simulink model "filterbankFIRFINALNOCOMP"  (R2018a)
settings: Solver=FixedStepDiscrete  StartTime=0.0  StopTime=0.001  RelTol=1e-3
values from neighbouring files (symbols this model uses):
  fs = 20000    [filterbankProto.m]    (also in main.m = 44100)
  gainConsts = 10.^(requiredGainDB/10)    [main.m]
undefined symbols (not defined in the file or in its folder): fdesignblkfcn, gcbh
libraries: dspsrcs4 x1, dspxfrm3 x1, dspobslib x1
(part 1 of 3)
settings Model: SimulationMode=accelerator  Creator=Kavi  LastModifiedBy=Kavi
settings SolverCC: AutoInsertRateTranBlk=on
settings DataIOCC: LimitDataPoints=on  SaveOutput=off  SignalLogging=off  SaveTime=off
settings OptimizationCC: LifeSpan=inf  SimCompilerOptimization=on
settings DebuggingCC: AlgebraicLoopMsg=error  SingleTaskRateTransMsg=error  AllowSymbolicDim=off  SFUnexpectedBacktrackingDiag=warning  SFNoUnconditionalDefaultTransitionDiag=warning  SFExecutionAtInitializationDiag=none
settings CodeAppCC: StateflowObjectComments=on
settings GRTTargetCC: TargetLangStandard=C89/C90 (ANSI)  GeneratePreprocessorConditionals=Disable all
settings ConfigComp: CovMetricSettings=dw  CovHtmlReporting=on  CovSaveCumulativeToWorkspaceVar=on  CovSaveSingleToWorkspaceVar=on  CovExternalEMLEnable=off  CovSFcnEnable=off

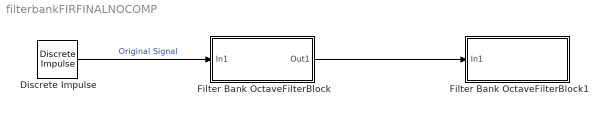
== system filterbankFIRFINALNOCOMP ==
  Discrete Impulse : dspsrcs4/Discrete  Impulse  Delay=0  SampleTime=1/fs  FrameSample=512  OutputFrames=off  dataType=double  isSigned=on  wordLen=16  udDataType=sfix(16)  fracBitsMode=Best precision  numFracBits=15  OutDataTypeStr=double  LastOutDataTypeStr=double
  Filter Bank OctaveFilterBlock : Subsystem
  Filter Bank OctaveFilterBlock1 : Subsystem
  wires:
  Discrete Impulse/1 -> Filter Bank OctaveFilterBlock/1(In1)  "Original Signal"
  Filter Bank OctaveFilterBlock/1(Out1) -> Filter Bank OctaveFilterBlock1/1(In1)

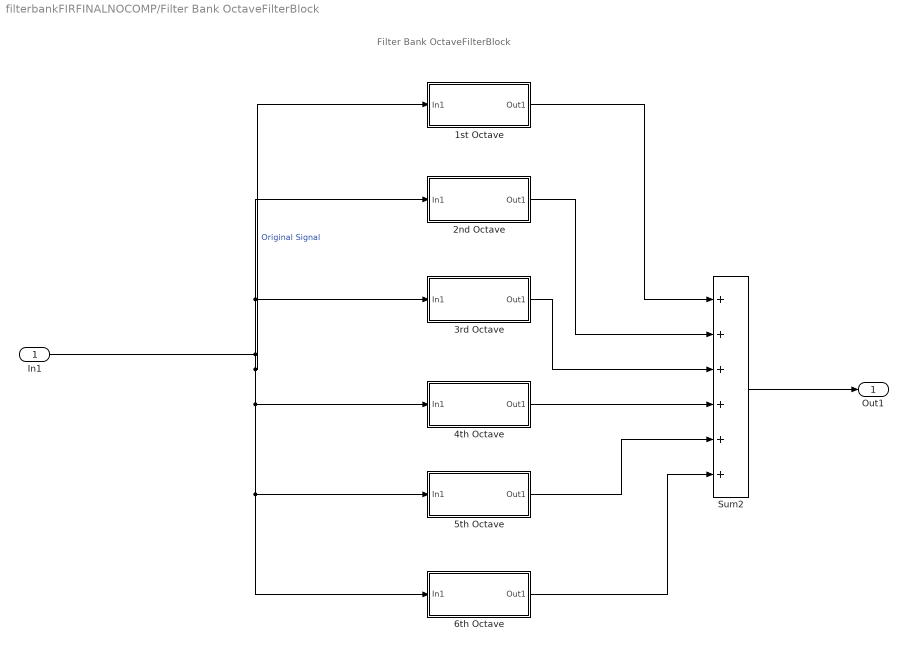
== system filterbankFIRFINALNOCOMP/Filter Bank OctaveFilterBlock ==
  note: Filter Bank OctaveFilterBlock
  In1 : Inport
  "1st Octave " : Subsystem
  2nd Octave : Subsystem
  "3rd Octave " : Subsystem
  4th Octave : Subsystem
  5th Octave : Subsystem
  6th Octave : Subsystem
  Sum2 : Sum  Inputs=++++++
  Out1 : Outport
  wires:
  Sum2/1 -> Out1/1
  2nd Octave/1(Out1) -> Sum2/2
  "3rd Octave "/1(Out1) -> Sum2/3
  4th Octave/1(Out1) -> Sum2/4
  5th Octave/1(Out1) -> Sum2/5
  6th Octave/1(Out1) -> Sum2/6
  In1/1 -> 4th Octave/1(In1), 5th Octave/1(In1), 6th Octave/1(In1), "1st Octave "/1(In1), "3rd Octave "/1(In1), 2nd Octave/1(In1)  "Original Signal"
  "1st Octave "/1(Out1) -> Sum2/1

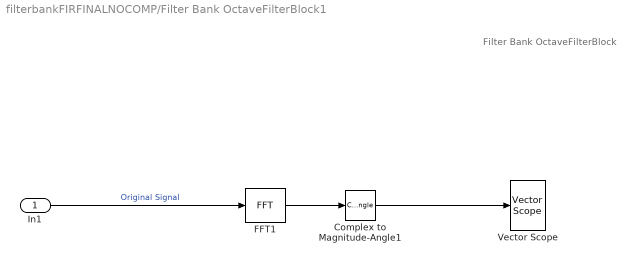
== system filterbankFIRFINALNOCOMP/Filter Bank OctaveFilterBlock1 ==
  note: Filter Bank OctaveFilterBlock
  In1 : Inport
  Complex to Magnitude-Angle1 : ComplexToMagnitudeAngle  Output=Magnitude
  FFT1 : dspxfrm3/FFT  FFTImplementation=Auto  CompMethod=Table lookup  TableOpt=NEW  TableOptActive=Speed  BitRevOrder=off  Normalize=off  InheritFFTLength=on  FFTLength=64  WrapInput=on  roundingMode=Floor  overflowMode=off  firstCoeffDataTypeStr=Inherit: Same word length as input  firstCoeffLastDataTypeStr=Inherit: Same word length as input  outputMin=[]  outputMax=[]
  Vector Scope : dspobslib/Vector Scope  ScopeProperties=off  Domain=Frequency  HorizSpan=1  DisplayProperties=off  AxisGrid=on  Memory=off  FrameNumber=on  AxisLegend=off  AxisZoom=off  OpenScopeAtSimStart=on  OpenScopeImmediately=off  FigPos=[86 244 1118 420]  AxisProperties=on  XUnits=Hertz  XRange=[0...Fs/2]  InheritXIncr=on  XIncr=1  XLabel=Samples  XLimit=Auto  XMin=0  XMax=1  XStart=0  YUnits=dB  YLabel=|Magnitude (dB)|  LineProperties=off  LineStyles=-  LineMarkers=None  LineColors=[0 0 0]  XAxisParamsVer=6.9
      settings: SourceProductName=DSP System Toolbox  SourceProductBaseCode=DS  YMin=0.0723692553519949  YMax=69.3188381671759
  wires:
  Complex to Magnitude-Angle1/1 -> Vector Scope/1
  FFT1/1 -> Complex to Magnitude-Angle1/1
  In1/1 -> FFT1/1  "Original Signal"

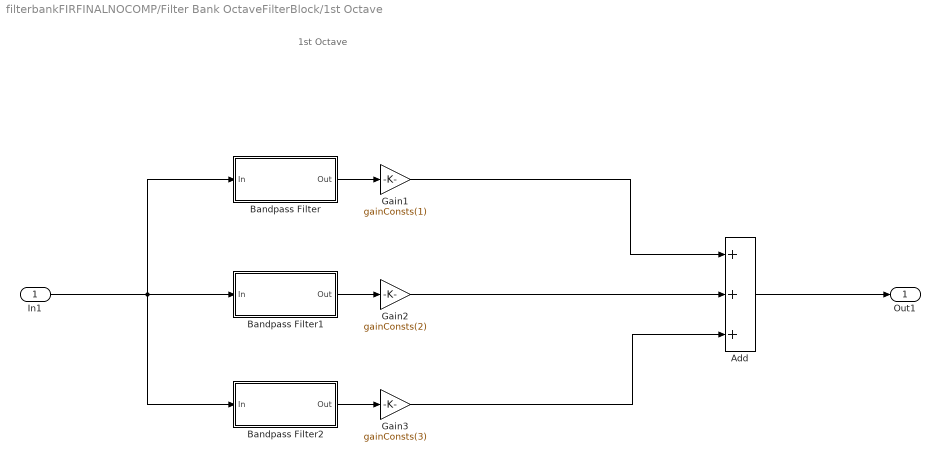
== system filterbankFIRFINALNOCOMP/Filter Bank OctaveFilterBlock/1st Octave  ==
  note: 1st Octave
  In1 : Inport
  Add : Sum  Inputs=+++
  Bandpass Filter : Subsystem  DialogController=fdesignblkfcn  InitFcn=fdesignblkfcn(gcbh, {'InitFcn'});  mask(Bandpass Filter){}
      mask help: Design a bandpass filter
      settings: CopyFcn=fdesignblkfcn(gcbh, {'CopyFcn'});
      mask Help: helpview(mapfilelocation('dsp'), 'dspbandpassfilter');
      mask Display: disp('Bandpass');
  Bandpass Filter1 : Subsystem  DialogController=fdesignblkfcn  InitFcn=fdesignblkfcn(gcbh, {'InitFcn'});  mask(Bandpass Filter){}
      mask help: Design a bandpass filter
      settings: CopyFcn=fdesignblkfcn(gcbh, {'CopyFcn'});
      mask Help: helpview(mapfilelocation('dsp'), 'dspbandpassfilter');
      mask Display: disp('Bandpass');
  Bandpass Filter2 : Subsystem  DialogController=fdesignblkfcn  InitFcn=fdesignblkfcn(gcbh, {'InitFcn'});  mask(Bandpass Filter){}
      mask help: Design a bandpass filter
      settings: CopyFcn=fdesignblkfcn(gcbh, {'CopyFcn'});
      mask Help: helpview(mapfilelocation('dsp'), 'dspbandpassfilter');
      mask Display: disp('Bandpass');
  Gain1 : Gain  Gain=gainConsts(1)
  Gain2 : Gain  Gain=gainConsts(2)
  Gain3 : Gain  Gain=gainConsts(3)
  Out1 : Outport
  wires:
  Bandpass Filter1/1(Out) -> Gain2/1
  Bandpass Filter2/1(Out) -> Gain3/1
  Add/1 -> Out1/1
  In1/1 -> Bandpass Filter/1(In), Bandpass Filter2/1(In), Bandpass Filter1/1(In)
  Bandpass Filter/1(Out) -> Gain1/1
  Gain1/1 -> Add/1
  Gain2/1 -> Add/2
  Gain3/1 -> Add/3

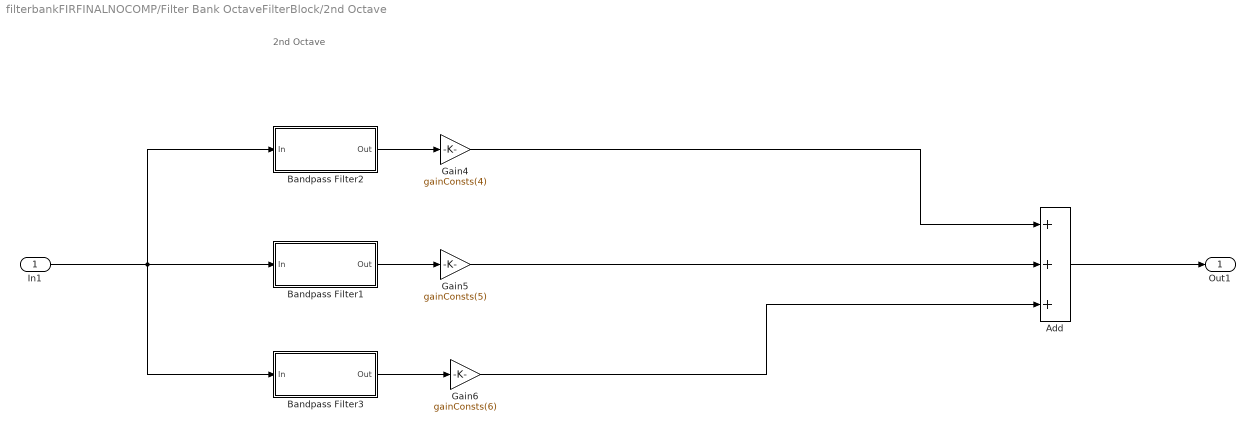
== system filterbankFIRFINALNOCOMP/Filter Bank OctaveFilterBlock/2nd Octave ==
  note: 2nd Octave
  In1 : Inport
  Add : Sum  Inputs=+++
  Bandpass Filter1 : Subsystem  DialogController=fdesignblkfcn  InitFcn=fdesignblkfcn(gcbh, {'InitFcn'});  mask(Bandpass Filter){}
      mask help: Design a bandpass filter
      settings: CopyFcn=fdesignblkfcn(gcbh, {'CopyFcn'});
      mask Help: helpview(mapfilelocation('dsp'), 'dspbandpassfilter');
      mask Display: disp('Bandpass');
  Bandpass Filter2 : Subsystem  DialogController=fdesignblkfcn  InitFcn=fdesignblkfcn(gcbh, {'InitFcn'});  mask(Bandpass Filter){}
      mask help: Design a bandpass filter
      settings: CopyFcn=fdesignblkfcn(gcbh, {'CopyFcn'});
      mask Help: helpview(mapfilelocation('dsp'), 'dspbandpassfilter');
      mask Display: disp('Bandpass');
  Bandpass Filter3 : Subsystem  DialogController=fdesignblkfcn  InitFcn=fdesignblkfcn(gcbh, {'InitFcn'});  mask(Bandpass Filter){}
      mask help: Design a bandpass filter
      settings: CopyFcn=fdesignblkfcn(gcbh, {'CopyFcn'});
      mask Help: helpview(mapfilelocation('dsp'), 'dspbandpassfilter');
      mask Display: disp('Bandpass');
  Gain4 : Gain  Gain=gainConsts(4)
  Gain5 : Gain  Gain=gainConsts(5)
  Gain6 : Gain  Gain=gainConsts(6)
  Out1 : Outport
  wires:
  In1/1 -> Bandpass Filter3/1(In), Bandpass Filter1/1(In), Bandpass Filter2/1(In)
  Bandpass Filter1/1(Out) -> Gain5/1
  Bandpass Filter2/1(Out) -> Gain4/1
  Bandpass Filter3/1(Out) -> Gain6/1
  Add/1 -> Out1/1
  Gain4/1 -> Add/1
  Gain5/1 -> Add/2
  Gain6/1 -> Add/3

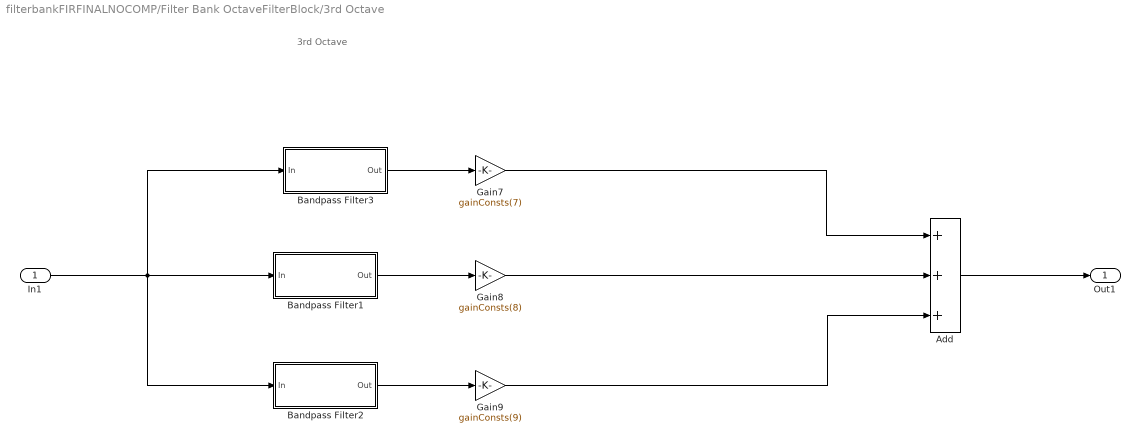
== system filterbankFIRFINALNOCOMP/Filter Bank OctaveFilterBlock/3rd Octave  ==
  note: 3rd Octave
  In1 : Inport
  Add : Sum  Inputs=+++
  Bandpass Filter1 : Subsystem  DialogController=fdesignblkfcn  InitFcn=fdesignblkfcn(gcbh, {'InitFcn'});  mask(Bandpass Filter){}
      mask help: Design a bandpass filter
      settings: CopyFcn=fdesignblkfcn(gcbh, {'CopyFcn'});
      mask Help: helpview(mapfilelocation('dsp'), 'dspbandpassfilter');
      mask Display: disp('Bandpass');
  Bandpass Filter2 : Subsystem  DialogController=fdesignblkfcn  InitFcn=fdesignblkfcn(gcbh, {'InitFcn'});  mask(Bandpass Filter){}
      mask help: Design a bandpass filter
      settings: CopyFcn=fdesignblkfcn(gcbh, {'CopyFcn'});
      mask Help: helpview(mapfilelocation('dsp'), 'dspbandpassfilter');
      mask Display: disp('Bandpass');
  Bandpass Filter3 : Subsystem  DialogController=fdesignblkfcn  InitFcn=fdesignblkfcn(gcbh, {'InitFcn'});  mask(Bandpass Filter){}
      mask help: Design a bandpass filter
      settings: CopyFcn=fdesignblkfcn(gcbh, {'CopyFcn'});
      mask Help: helpview(mapfilelocation('dsp'), 'dspbandpassfilter');
      mask Display: disp('Bandpass');
  Gain7 : Gain  Gain=gainConsts(7)
  Gain8 : Gain  Gain=gainConsts(8)
  Gain9 : Gain  Gain=gainConsts(9)
  Out1 : Outport
  wires:
  In1/1 -> Bandpass Filter2/1(In), Bandpass Filter1/1(In), Bandpass Filter3/1(In)
  Bandpass Filter1/1(Out) -> Gain8/1
  Bandpass Filter3/1(Out) -> Gain7/1
  Bandpass Filter2/1(Out) -> Gain9/1
  Add/1 -> Out1/1
  Gain7/1 -> Add/1
  Gain8/1 -> Add/2
  Gain9/1 -> Add/3

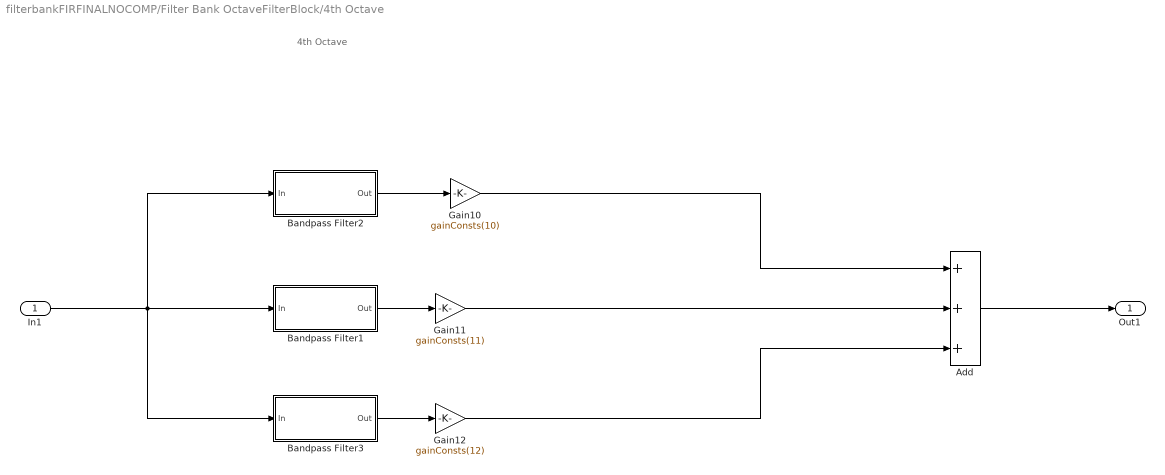
== system filterbankFIRFINALNOCOMP/Filter Bank OctaveFilterBlock/4th Octave ==
  note: 4th Octave
  In1 : Inport
  Add : Sum  Inputs=+++
  Bandpass Filter1 : Subsystem  DialogController=fdesignblkfcn  InitFcn=fdesignblkfcn(gcbh, {'InitFcn'});  mask(Bandpass Filter){}
      mask help: Design a bandpass filter
      settings: CopyFcn=fdesignblkfcn(gcbh, {'CopyFcn'});
      mask Help: helpview(mapfilelocation('dsp'), 'dspbandpassfilter');
      mask Display: disp('Bandpass');
  Bandpass Filter2 : Subsystem  DialogController=fdesignblkfcn  InitFcn=fdesignblkfcn(gcbh, {'InitFcn'});  mask(Bandpass Filter){}
      mask help: Design a bandpass filter
      settings: CopyFcn=fdesignblkfcn(gcbh, {'CopyFcn'});
      mask Help: helpview(mapfilelocation('dsp'), 'dspbandpassfilter');
      mask Display: disp('Bandpass');
  Bandpass Filter3 : Subsystem  DialogController=fdesignblkfcn  InitFcn=fdesignblkfcn(gcbh, {'InitFcn'});  mask(Bandpass Filter){}
      mask help: Design a bandpass filter
      settings: CopyFcn=fdesignblkfcn(gcbh, {'CopyFcn'});
      mask Help: helpview(mapfilelocation('dsp'), 'dspbandpassfilter');
      mask Display: disp('Bandpass');
  Gain10 : Gain  Gain=gainConsts(10)
  Gain11 : Gain  Gain=gainConsts(11)
  Gain12 : Gain  Gain=gainConsts(12)
  Out1 : Outport
  wires:
  In1/1 -> Bandpass Filter3/1(In), Bandpass Filter1/1(In), Bandpass Filter2/1(In)
  Bandpass Filter1/1(Out) -> Gain11/1
  Bandpass Filter2/1(Out) -> Gain10/1
  Bandpass Filter3/1(Out) -> Gain12/1
  Add/1 -> Out1/1
  Gain10/1 -> Add/1
  Gain11/1 -> Add/2
  Gain12/1 -> Add/3

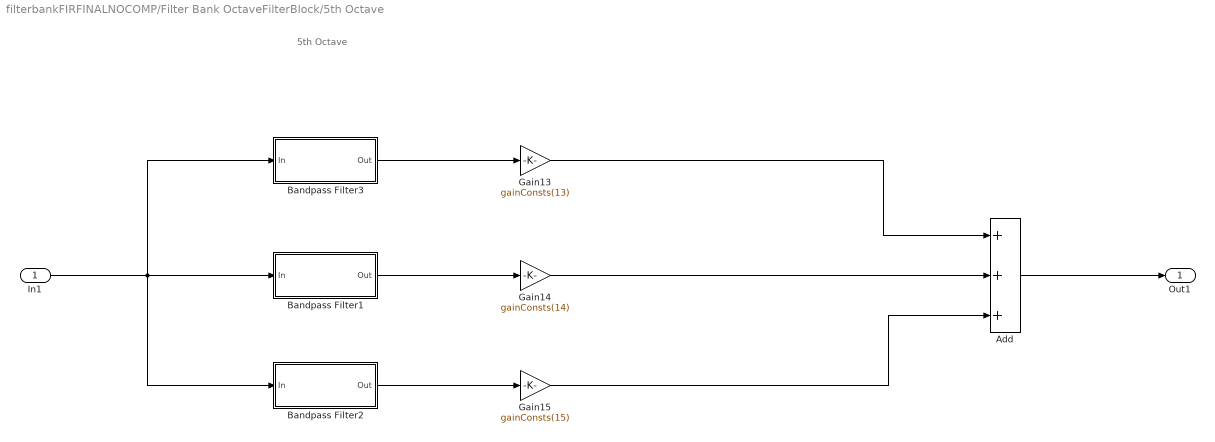
== system filterbankFIRFINALNOCOMP/Filter Bank OctaveFilterBlock/5th Octave ==
  note: 5th Octave
  In1 : Inport
  Add : Sum  Inputs=+++
  Bandpass Filter1 : Subsystem  DialogController=fdesignblkfcn  InitFcn=fdesignblkfcn(gcbh, {'InitFcn'});  mask(Bandpass Filter){}
      mask help: Design a bandpass filter
      settings: CopyFcn=fdesignblkfcn(gcbh, {'CopyFcn'});
      mask Help: helpview(mapfilelocation('dsp'), 'dspbandpassfilter');
      mask Display: disp('Bandpass');
  Bandpass Filter2 : Subsystem  DialogController=fdesignblkfcn  InitFcn=fdesignblkfcn(gcbh, {'InitFcn'});  mask(Bandpass Filter){}
      mask help: Design a bandpass filter
      settings: CopyFcn=fdesignblkfcn(gcbh, {'CopyFcn'});
      mask Help: helpview(mapfilelocation('dsp'), 'dspbandpassfilter');
      mask Display: disp('Bandpass');
  Bandpass Filter3 : Subsystem  DialogController=fdesignblkfcn  InitFcn=fdesignblkfcn(gcbh, {'InitFcn'});  mask(Bandpass Filter){}
      mask help: Design a bandpass filter
      settings: CopyFcn=fdesignblkfcn(gcbh, {'CopyFcn'});
      mask Help: helpview(mapfilelocation('dsp'), 'dspbandpassfilter');
      mask Display: disp('Bandpass');
  "Gain13 " : Gain  Gain=gainConsts(13)
  Gain14 : Gain  Gain=gainConsts(14)
  Gain15 : Gain  Gain=gainConsts(15)
  Out1 : Outport
  wires:
  In1/1 -> Bandpass Filter2/1(In), Bandpass Filter1/1(In), Bandpass Filter3/1(In)
  Bandpass Filter1/1(Out) -> Gain14/1
  Bandpass Filter3/1(Out) -> "Gain13 "/1
  Bandpass Filter2/1(Out) -> Gain15/1
  Add/1 -> Out1/1
  "Gain13 "/1 -> Add/1
  Gain14/1 -> Add/2
  Gain15/1 -> Add/3

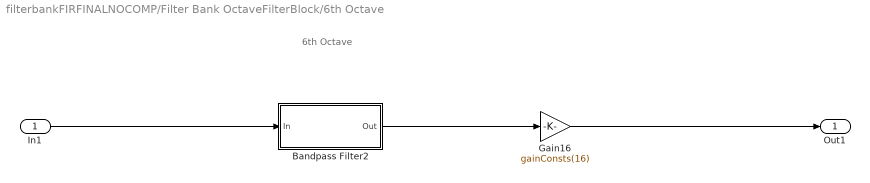
== system filterbankFIRFINALNOCOMP/Filter Bank OctaveFilterBlock/6th Octave ==
  note: 6th Octave
  In1 : Inport
  Bandpass Filter2 : Subsystem  DialogController=fdesignblkfcn  InitFcn=fdesignblkfcn(gcbh, {'InitFcn'});  mask(Bandpass Filter){}
      mask help: Design a bandpass filter
      settings: CopyFcn=fdesignblkfcn(gcbh, {'CopyFcn'});
      mask Help: helpview(mapfilelocation('dsp'), 'dspbandpassfilter');
      mask Display: disp('Bandpass');
  Gain16 : Gain  Gain=gainConsts(16)
  Out1 : Outport
  wires:
  In1/1 -> Bandpass Filter2/1(In)
  Bandpass Filter2/1(Out) -> Gain16/1
  Gain16/1 -> Out1/1

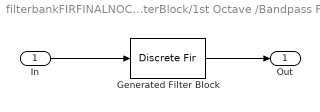
== system filterbankFIRFINALNOCOMP/Filter Bank OctaveFilterBlock/1st Octave /Bandpass Filter ==
  In : Inport
  Generated Filter Block : DiscreteFir  Tag=BlockMethodSubSystem  Coefficients=[0.00069254263564703239 7.08332125616228079e-05 7.43338221660424489e-05 7.78019514310851305e-05 8.1313055894969587e-05 8.47676145299332306e-05 8.82427360820155573e-05 9.16321724960766058e-05 9.50132779449859897e-05 9.82780844645089513e-05 0.000101505416215626917 0.000104588272515063408 0.000107617215710334275 0.00011047625362861513 0.00011327190922524107 0.00011588720344087749 0.000118439063772244506 0.000120801645064717676 0.000123099948028595888 0.000125185473013980539 0.000127187073587639766 0.000128920397422576543 0.000130511390648946173 0.000131743702029481316 0.000132780552104568809 0.000133389417172361956 0.000133854650892706686 0.000133962102161934026 0.000134191447940623887 0.000134157907401536596 0.000134265802405980015 0.000131964127362239067 0.000131332829006028655 0.000129881713135985254 0.000127781891228210658 0.00012560624825513878 0.000122871669998617469 0.000119905227728997496 0.000116437763341584356 0.000112673160055361417 0.000108423322441774915 0.000103831634900475322 9.87550170397490595e-05 9.32921756593519465e-05 8.73418076823880148e-05 8.09793421469050311e-05 7.41320849184379238e-05 6.68640900405536692e-05 5.91280126399577657e-05 5.09709728131291259e-05 4.23580286976533879e-05 3.33043823994830487e-05 2.37740038396172157e-05 1.37639365669146765e-05 3.26127779076603809e-06 -7.7317453512068843e-06 -1.91529644642969859e-05 -3.10003177523197578e-05 -4.31932861316397014e-05 -5.58837065186529896e-05 -6.90579370056025566e-05 -8.29329326828186165e-05 -9.66811793280690957e-05 -0.000111145779536190516 -0.00012609897719820774 -0.000141236461222010983 -0.000156929308144654366 -0.000172865242278997746 -0.000189252021719758069 -0.000205888412220562174 -0.000222913900982208096 -0.000240171049308351715 -0.000257771369782683487 -0.000275586047472969214 -0.000293697318135855215 -0.000311995161659652973 -0.000330540765463578038 -0.000349224903827191667 -0.000368090528662009197 -0.000387036436696074917 -0.000406100594965500266 -0.000425203831895935142 -0.000444384091535106568 -0.000463566273616394841 -0.000482772030573579819 -0.000501910732114202863 -0.000520965897608973881 -0.000539873027512084366 -0.000558637930834297728 -0.000577262628276531539 -0.000595709307139574988 -0.000613892477578554282 -0.000631638639673933518 -0.000649243044828252632 -0.000666485727740266675 -0.000683200994276255205 -0.000699649189317232243 -0.000715512234643985627 -0.000730963186339991995 -0.000745795559867745207 -0.000760109236317694603 -0.000773741289031793173 -0.000786770921834983135 -0.000799056123573673566 -0.000810658888349138408 -0.000821455874060750225 -0.000831492219624249316 -0.000840644134899665857 -0.000848948904248300672 -0.000856290612773433885 -0.000862709405070977002 -0.000868105460333159704 -0.000872517740327855939 -0.000875845912368163212 -0.000878119868504033678 -0.000879228408584138872 -0.000879197077001071282 -0.000877952246535155341 -0.000875532061713544477 -0.00087186975855863371 -0.000866948352418330068 -0.000860675447894846627 -0.000853080747161018152 -0.000844214330725798667 -0.000833949246744723999 -0.000822227747335713089 -0.000809237906740421981 -0.000794711847269004117 -0.000778841968040845461 -0.000761455634202649239 -0.000742666062579664223 -0.000722354149934576286 -0.000700615104156640371 -0.000677349389871262386 -0.000652647074842618987 -0.000626425686320928698 -0.000598762403763111782 -0.000569579411754098336 -0.000538956905907554207 -0.000506826531392092156 -0.000473276746412924592 -0.000438250037486827011 -0.000401833809678808578 -0.000363970583238830685 -0.000324746531243159215 -0.000284103795984386219 -0.000242145735403713139 -0.000198843759525243812 -0.000154293216207523979 -0.000108454831747326099 -6.14002678822141477e-05 -1.31139495230440297e-05 3.62779841181725719e-05 8.6783675707447622e-05 0.000138378871254365727 0.00019102420818066271 0.000244546823067770189 0.000299100706116297167 0.000354434756272426399 0.000410649716103439911 0.000467573009587186558 0.000525241288960216291 0.000583505567682658264 ...(+15055 chars)]  InputProcessing=Columns as channels (frame based)
  Out : Outport
  wires:
  In/1 -> Generated Filter Block/1
  Generated Filter Block/1 -> Out/1

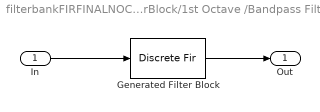
== system filterbankFIRFINALNOCOMP/Filter Bank OctaveFilterBlock/1st Octave /Bandpass Filter1 ==
  In : Inport
  Generated Filter Block : DiscreteFir  Tag=BlockMethodSubSystem  Coefficients=[0.000700210960206121584 9.08999096462534753e-05 9.6493475997903649e-05 0.000102024349867572018 0.000107612579626240111 0.000113115900856586922 0.000118635157897549709 0.000123976371066557181 0.000129207962104145699 0.000134098413991073332 0.000138779649990945731 0.000143130230806684847 0.000147557040668118704 0.000152034630484060144 0.000156719067589813346 0.000158909825070414706 0.000162726008646865749 0.000165461809806520012 0.000167783855788171247 0.000169746562233939985 0.000171215411686888959 0.000172200136269324774 0.000172609162236851666 0.000172384750360795994 0.000171519173262836772 0.000170020862647419536 0.000167999170775735731 0.000165344145247176911 0.000161919617694286514 0.000157405174630295035 0.00015271792888284176 0.000146845399392119685 0.000140266770773409401 0.000132911201673273339 0.000124688234048694348 0.000115633765799201906 0.000105661777361271223 9.47662932504614915e-05 8.29432590447714549e-05 7.0227563862974721e-05 5.66438152552955565e-05 4.21085238605347148e-05 2.658236253174739e-05 1.00801588851100231e-05 -7.14257405372655842e-06 -2.55393907655513059e-05 -4.47228028834414492e-05 -6.4799154773648583e-05 -8.5774760830036826e-05 -0.000107582385953470193 -0.000130268493930503168 -0.000153776316081986105 -0.000178077446118537629 -0.000203106206034891937 -0.000228843038064305347 -0.000255293770480404815 -0.000282406815516756575 -0.000310101255612749301 -0.000338299754500146247 -0.000367148359093456714 -0.000396334365821387861 -0.000425945836579554385 -0.000455901234348218007 -0.000486107662720235189 -0.000516560515447010054 -0.000547143766887328749 -0.000577796431113751356 -0.000608420122651499233 -0.000638964627698719611 -0.000669355850793235509 -0.000699488497864776812 -0.000729266037357153727 -0.000758630721857012362 -0.000787547623134470767 -0.000815774397095867486 -0.00084335280250142741 -0.000870136616413438174 -0.000896027159315731592 -0.000920976763761805427 -0.000944838854910358904 -0.000967543342301744637 -0.000988976439555649825 -0.00100906814852505826 -0.00102770542898750943 -0.00104478372064510531 -0.00106021709472175043 -0.0010739404283370941 -0.00108585069345779354 -0.00109578977675205765 -0.0011037686753822668 -0.00110963346832027108 -0.00111331859885226234 -0.00111476979672931733 -0.00111386123676532377 -0.00111055540660976717 -0.00110475906574658556 -0.00109642442186392154 -0.00108546184900020848 -0.00107182088550054747 -0.0010554590512113981 -0.00103633765031815915 -0.00101438430436361104 -0.000989547634722831929 -0.000961851003137375454 -0.000931204573781415864 -0.000897620079413248236 -0.000861089001791935193 -0.0008215667004735685 -0.000779092867196282558 -0.00073364243816827733 -0.000685243230312603067 -0.000633889786258891221 -0.000579629348660391482 -0.00052249816622848555 -0.000462536609697427519 -0.000399771065553664918 -0.000334272977530827051 -0.00026612493320221837 -0.000195354826563743571 -0.000122080355274795907 -4.63788968579434023e-05 3.16732415595984617e-05 0.000111935744140494739 0.000194335110415129637 0.000278734735218747636 0.00036502978398468295 0.000453062491483400588 0.000542703929883438328 0.000633809806648881089 0.000726238185418645859 0.000819809817723408853 0.000914365859188095878 0.00100975644434884299 0.00110577180710032361 0.00120224808729774927 0.00129900003352437666 0.00139580723292306625 0.00149251086466925639 0.00158888338826579574 0.00168473694169961807 0.0017798388729062301 0.00187399500203089438 0.00196698598924061269 0.00205859787931057629 0.0021485975095779028 0.00223678264607570995 0.00232293388755837674 0.00240681073733488727 0.00248821177642774907 0.00256690855965325832 0.0026426689803898621 0.00271530927911167166 0.00278458430729308691 0.00285030157149111394 0.00291223291154696189 0.0029701938039841066 0.00302397088021196751 0.00307337191464770575 0.00311819915855655969 0.00315828646704071399 0.00319344503317399225 0.0032234982496808103 0.00324829691310643889 0.00326767215413426406 0.0032814770042531396 0.00328959626736713504 ...(+11094 chars)]  InputProcessing=Columns as channels (frame based)
  Out : Outport
  wires:
  In/1 -> Generated Filter Block/1
  Generated Filter Block/1 -> Out/1
